simulink model "metareasoning"  (R2020a)
settings: Solver=FixedStepAuto  StartTime=0.0  StopTime=1000  FixedStep=0.5  RelTol=1e-3
PreLoadFcn:
  | Metareasoningpreloadfcn
InitFcn:
  | MetareasoningInitFcn
StopFcn:
  | trajectory_plot
values from neighbouring files (symbols this model uses):
  Clmax = 2.0    (= 2)    [Metareasoningpreloadfcn.m]
  Clmin = -.5    (= -0.5)    [Metareasoningpreloadfcn.m]
  g = 9.81    [Metareasoningpreloadfcn.m]
  goal_pos = [9000, 1E6, 0; -1E6, 23150+9000, 0]    [MetareasoningInitFcn.m]
  LOS_m = 9260    [Metareasoningpreloadfcn.m]
  num_ac = 2    [MetareasoningInitFcn.m]
  omega_chi = .2    (= 0.2)    [Metareasoningpreloadfcn.m]
  omega_gamma = .2    (= 0.2)    [Metareasoningpreloadfcn.m]
  omega_v = .3    (= 0.3)    [Metareasoningpreloadfcn.m]
  rho = 1.225    [Metareasoningpreloadfcn.m]
  S = 37.161    [Metareasoningpreloadfcn.m]
  tau_b = .5    (= 0.5)    [Metareasoningpreloadfcn.m]
  tau_n = .5    (= 0.5)    [Metareasoningpreloadfcn.m]
  tau_t = 1    [Metareasoningpreloadfcn.m]
  thrust_ic = 0.5*rho.*vel_ic.^2*S.*Cd    [MetareasoningInitFcn.m]
  Tmax = 25600*4.44822    (= 113874.432)    [Metareasoningpreloadfcn.m]
  W = 14515    [Metareasoningpreloadfcn.m]
undefined symbols (not defined in the file or in its folder): turnangles
libraries: asbswarm_lib x2, aerolibptmass x2, simulink x1
(part 3 of 3)

== matlab function metareasoning/Conflict Resolution/Erzberger 2010/Cooperative Maneuvers/A Right B Left/Find Resolution ==
  data: x input; type output; y input; V input; chi input; dt input; tt input; R input; angles input; resangle output; restime output; minsep output; dt_min output; tt_min output; dphi_min output
function [type, resangle, restime, minsep, dt_min, tt_min, dphi_min] = A_right_B_left(x,y, V, chi, dt, tt, R, angles)
    
    xa0 = x(1);
    xb0 = x(2);
    ya0 = y(1);
    yb0 = y(2);
    va = V(1);
    vb = V(2);
    hdgb = chi(2);
    hdga = chi(1);
    Ra = R(1);
    Rb = R(2);
    taa = angles;
    tab = -abs(va./vb./angles);
    LOS_m = 9260;
    
    % turn parameters
    [dt_min, idx] = min(dt);
    tt_min = tt(idx);
    dphi_min = angles(idx);
    
    % eqn.6
    xa1 = Ra.*sign(taa).* (1-cos(taa));
    ya1 = Ra.*sign(taa).* sin(taa);
    
    % eqn.8
    xb1 = xb0 + Rb.*sign(tab).*cos(hdgb) - Rb.*sign(tab).*cos(hdgb + angles);
    yb1 = yb0 - Rb.*sign(tab).*sin(hdgb) + Rb.*sign(tab).*sin(hdgb + angles);
    
    % eqn.17
    dx1 = xb1 - xa1;
    dy1 = yb1 - ya1;
    vrx = vb.*sin(hdgb+tab) - va.*sin(hdga+taa);
    vry = vb.*cos(hdgb+tab) - va.*cos(hdga+taa);
    
    % eqn.18
    vrsq = vrx.^2 + vry.^2;
    ts_min = -(dx1.*vrx + dy1.*vry)./vrsq;
    
    % eqn. 19
    foo = dx1.*vrx + dy1.*vry;
    bar1 = dx1 - vrx.*foo./vrsq;
    bar2 = dy1 - vry.*foo./vrsq;
    ds_min = sqrt(bar1.^2 + bar2.^2);
    
    % execution times
    ts_min(ts_min < 0) = 0; % set negative values = 0
    t_exec = tt + ts_min;
    
    % find resolution
    
    %fake res parameters
    type = 2;
    resangle = 0;
    restime = 0;
    minsep = 0;
    residx = 1;
    
    %[skipping weird maxima stuff]
    
    % check for type 1
    if dt_min >= LOS_m
        type = 1;
        for i = 1:length(ds_min)
            if ds_min(i) >= LOS_m
                residx = i;
                break
            end
        end
        minsep = ds_min(residx);
        resangle = angles(residx);
        restime = t_exec(residx);
        % check for 1a
        if restime > 1.2 * tt_min
            type = 1.1;
            minsep = dt_min;
            resangle = dphi_min;
            restime = tt_min;
        end
    end   
end

== matlab function metareasoning/Conflict Detection/State-Based Conflict Detection (Single Agent)/Detect Conflict for Each Intruder/Conflict Detection ==
  data: v_own input; tlos output; x_own input; v_int input; x_int input; tcpa output; LOS_m input
function [tlos, tcpa] = statebasedCD(v_own, x_own, v_int, x_int, LOS_m)
% BlueSky on GitHub, ASAS- CD&R-info.pdf 

    R = LOS_m;
    
    v_rel = v_own - v_int;
    x_rel = x_int - x_own;
    
    if v_rel(1) == 0 && v_rel(2) == 0
        tlos = NaN;
        tcpa = NaN;
    else
        poly = [dot(v_rel,v_rel), -2*dot(x_rel,v_rel), dot(x_rel, x_rel) - R^2];
        tloses = roots(poly); 
        tlos = real(min(tloses)); % Time until loss of separation
        tcpa = dot(x_rel,v_rel)/dot(v_rel,v_rel); % Time of closest point of approach
    end
    
end

== matlab function metareasoning/Conflict Resolution/Frazzoli 2005 CR/Single-Agent Planning/Select State ==
  data: obs input; phi input; not_at_goal input; bank output; chi input; mu_roll input; mu_hold input; loadfactor output; min_free input
function [bank, loadfactor] = selectstate(obs, phi, not_at_goal, chi, mu_roll, mu_hold, min_free)
    bank = mu_hold;
    
    %Angle Differences
    goal_diff = phi - chi;
    obs_diff = min_free - chi;
    goal_diff = mod(goal_diff, 2*pi)
    obs_diff = mod(obs_diff, 2*pi)
   
    if (abs(goal_diff) <= 1*(pi/180) || abs(goal_diff) >= 358*(pi/180)) && not_at_goal == 1 && obs == 0
        bank = 0;
    end
%     if (abs(obs_diff) <= 2*(pi/180) || abs(goal_diff) >= 358*(pi/180)) && not_at_goal == 1 && obs == 1
%         bank = -mu_roll;
%     end
    loadfactor = 1/cos(bank);
    
end

== matlab function metareasoning/Conflict Resolution/Erzberger 2010/Standard Maneuvers/d_b (11)/Eqn. 10 ==
  data: Va input; db output; hdgb input; xb input; yb input; t input; Rb input
function db = fcn(Va, hdgb, xb, yb, t, Rb)
    turnangle = [-150:2:150].';
    turnangle = deg2rad(turnangle);
    q = (xb + Rb.*sign(turnangle).*cos(hdgb) - Rb.*sign(turnangle).*cos(hdgb + turnangle)).^2;
    r = (yb - t.*Va - Rb.*sign(turnangle).*sin(hdgb) + Rb.*sign(turnangle).*sin(hdgb + turnangle)).^2;
    db = sqrt(q + r);
end

== matlab function metareasoning/Conflict Resolution/Erzberger 2010/Standard Maneuvers/A Right B Straight/A_right_B_straight ==
  data: x input; type output; y input; V input; chi input; dt input; tt input; Ra input; angles input; resangle output; restime output; minsep output; dt_min output; tt_min output; dphi_min output
function [type, resangle, restime, minsep, dt_min, tt_min, dphi_min] = A_right_B_straight(x,y, V, chi, dt, tt, Ra, angles)
    
    xa0 = x(1);
    xb0 = x(2);
    ya0 = y(1);
    yb0 = y(2);
    va = V(1);
    vb = V(2);
    hdgb = chi(2);
    LOS_m = 9260;
    
    % eqn.6
    xa1 = Ra.*sign(angles).* (1-cos(angles));
    ya1 = Ra.*sign(angles).* sin(angles);
    
    % eqn.9
    xb1 = xb0 + tt.*vb.*sin(hdgb);
    yb1 = yb0 + tt.*vb.*cos(hdgb);
    
    % eqn.17
    dx1 = xb1 - xa1;
    dy1 = yb1 - ya1;
    vrx = vb.*sin(hdgb) - va.*sin(angles);
    vry = vb.*cos(hdgb) - va.*cos(angles);
    
    % eqn.18
    vrsq = vrx.^2 + vry.^2;
    ts_min = -(dx1.*vrx + dy1.*vry)./vrsq;
    
    % eqn. 19
    foo = dx1.*vrx + dy1.*vry;
    bar1 = dx1 - vrx.*foo./vrsq;
    bar2 = dy1 - vry.*foo./vrsq;
    ds_min = sqrt(bar1.^2 + bar2.^2);
    
    % execution times
    ts_min(ts_min < 0) = 0; % set negative values = 0
    t_exec = tt + ts_min;
    
    % turn parameters
    [dt_min, idx] = min(dt);
    tt_min = tt(idx);
    dphi_min = angles(idx);
    
    % find resolution
    %Fake res parameters
    type = 2;
    resangle = 0;
    restime = 0;
    minsep = 0;
    residx = 1;
    
    %[skipping weird maxima stuff]
    
    % check for type 1
    if dt_min >= LOS_m
        type = 1;
        for i = 1:length(ds_min)
            if ds_min(i) >= LOS_m
                residx = i;
                break
            end
        end
        minsep = ds_min(residx);
        resangle = angles(residx);
        restime = t_exec(residx);
        % check for 1a
        if restime > 1.2 * tt_min
            type = 1.1;
            minsep = dt_min;
            resangle = dphi_min;
            restime = tt_min;
        end
    end   
end

== matlab function metareasoning/Conflict Resolution/Erzberger 2010/Standard Maneuvers/A Left B Straight/A_left_B_straight ==
  data: x input; type output; y input; V input; chi input; dt input; tt input; Ra input; angles input; resangle output; restime output; minsep output; dt_min output; tt_min output; dphi_min output
function [type, resangle, restime, minsep, dt_min, tt_min, dphi_min] = A_left_B_straight(x,y, V, chi, dt, tt, Ra, angles)
    
    xa0 = x(1);
    xb0 = x(2);
    ya0 = y(1);
    yb0 = y(2);
    va = V(1);
    vb = V(2);
    hdgb = chi(2);
    LOS_m = 9260;
    
    % eqn.6
    xa1 = Ra.*sign(angles).* (1-cos(angles));
    ya1 = Ra.*sign(angles).* sin(angles);
    
    % eqn.9
    xb1 = xb0 + tt.*vb.*sin(hdgb);
    yb1 = yb0 + tt.*vb.*cos(hdgb);
    
    % eqn.17
    dx1 = xb1 - xa1;
    dy1 = yb1 - ya1;
    vrx = vb.*sin(hdgb) - va.*sin(angles);
    vry = vb.*cos(hdgb) - va.*cos(angles);
    
    % eqn.18
    vrsq = vrx.^2 + vry.^2;
    ts_min = -(dx1.*vrx + dy1.*vry)./vrsq;
    
    % eqn. 19
    foo = dx1.*vrx + dy1.*vry;
    bar1 = dx1 - vrx.*foo./vrsq;
    bar2 = dy1 - vry.*foo./vrsq;
    ds_min = sqrt(bar1.^2 + bar2.^2);
    
    % execution times
    ts_min(ts_min < 0) = 0; % set negative values = 0
    t_exec = tt + ts_min;
    
    % turn parameters
    [dt_min, idx] = min(dt);
    tt_min = tt(idx);
    dphi_min = angles(idx);
    
    % find resolution
    %Fake res parameters
    type = 2;
    resangle = 0;
    restime = 0;
    minsep = 0;
    residx = 1;
    
    %[skipping weird maxima stuff]
    
    % check for type 1
    if dt_min >= LOS_m
        type = 1;
        for i = length(ds_min):-1:1
            if ds_min(i) >= LOS_m
                residx = i;
                break
            end
        end
        minsep = ds_min(residx);
        resangle = angles(residx);
        restime = t_exec(residx);
        % check for 1a
        if restime > 1.2 * tt_min
            type = 1.1;
            minsep = dt_min;
            resangle = dphi_min;
            restime = tt_min;
        end
    end   
end

== matlab function metareasoning/Conflict Resolution/Erzberger 2010/Standard Maneuvers/A Straight B Left/Find Resolution ==
  data: x input; type output; y input; V input; chi input; dt input; tt input; Rb input; angles input; resangle output; restime output; minsep output; dt_min output; tt_min output; dphi_min output
function [type, resangle, restime, minsep, dt_min, tt_min, dphi_min] = A_straight_B_left(x,y, V, chi, dt, tt, Rb, angles)
    
    xa0 = x(1);
    xb0 = x(2);
    ya0 = y(1);
    yb0 = y(2);
    va = V(1);
    vb = V(2);
    hdgb = chi(2);
    hdga = chi(1);
    LOS_m = 9260;
    
    % eqn.8
    xb1 = xb0 + Rb.*sign(angles).*cos(hdgb) - Rb.*sign(angles).*cos(hdgb + angles);
    yb1 = yb0 - Rb.*sign(angles).*sin(hdgb) + Rb.*sign(angles).*sin(hdgb + angles);
    
    % a straight
    xa1 = xa0;
    ya1 = ya0 + va.*tt;
    
    % eqn.17
    dx1 = xb1 - xa1;
    dy1 = yb1 - ya1;
    vrx = vb.*sin(hdgb+angles) - va.*sin(hdga);
    vry = vb.*cos(hdgb+angles) - va.*cos(hdga);
    
    % eqn.18
    vrsq = vrx.^2 + vry.^2;
    ts_min = -(dx1.*vrx + dy1.*vry)./vrsq;
    
    % eqn. 19
    foo = dx1.*vrx + dy1.*vry;
    bar1 = dx1 - vrx.*foo./vrsq;
    bar2 = dy1 - vry.*foo./vrsq;
    ds_min = sqrt(bar1.^2 + bar2.^2);
    
    % execution times
    ts_min(ts_min < 0) = 0; % set negative values = 0
    t_exec = tt + ts_min;
    
    % turn parameters
    [dt_min, idx] = min(dt);
    tt_min = tt(idx);
    dphi_min = angles(idx);
    
    % find resolution
    
    %fake res parameters
    type = 2;
    resangle = 0;
    restime = 0;
    minsep = 0;
    residx = 1;
    
    %[skipping weird maxima stuff]
    
    % check for type 1
    if dt_min >= LOS_m
        type = 1;
        for i = length(ds_min):-1:1
            if ds_min(i) >= LOS_m
                residx = i;
                break
            end
        end
        minsep = ds_min(residx);
        resangle = angles(residx);
        restime = t_exec(residx);
        % check for 1a
        if restime > 1.2 * tt_min
            type = 1.1;
            minsep = dt_min;
            resangle = dphi_min;
            restime = tt_min;
        end
    end   
end
